simulink model "wheel_leg_backup_621"  (R2025b)
settings: Solver=VariableStepAuto  StartTime=0.0  StopTime=10  FixedStep=0.0001  RelTol=1e-3
undefined symbols (not defined in the file): g, M_L_support, X, Y, Z
libraries: sm_lib x76, nesl_utility x14, slpidlib x1
(part 1 of 3)
settings Model: PauseTimes=10  Creator=Hhop  LastModifiedBy=13422
settings SolverCC: AlgebraicLoopSolver=TrustRegion  MinimalZcImpactIntegration=on
settings DebuggingCC: ReadBeforeWriteMsg=DisableAll  WriteAfterWriteMsg=DisableAll  WriteAfterReadMsg=DisableAll  MultiTaskDSMMsg=none
settings ModelReferenceCC: UpdateModelReferenceTargets=IfOutOfDate
settings SFSimCC: SFSimEcho=off
settings RTWCC: GPUComputeCapability=3.5  DLArmComputeVersion=19.05

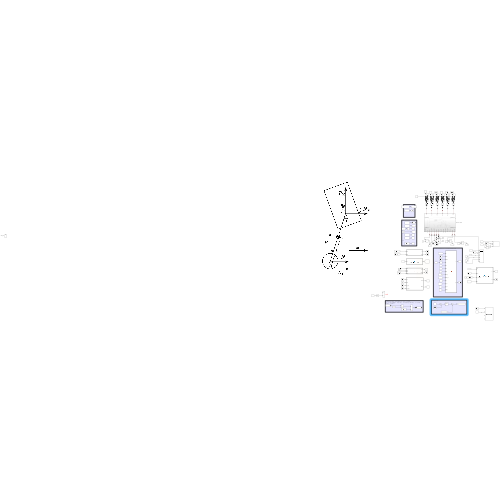
[thumbnail: Simulink's stored preview of the top-level diagram]
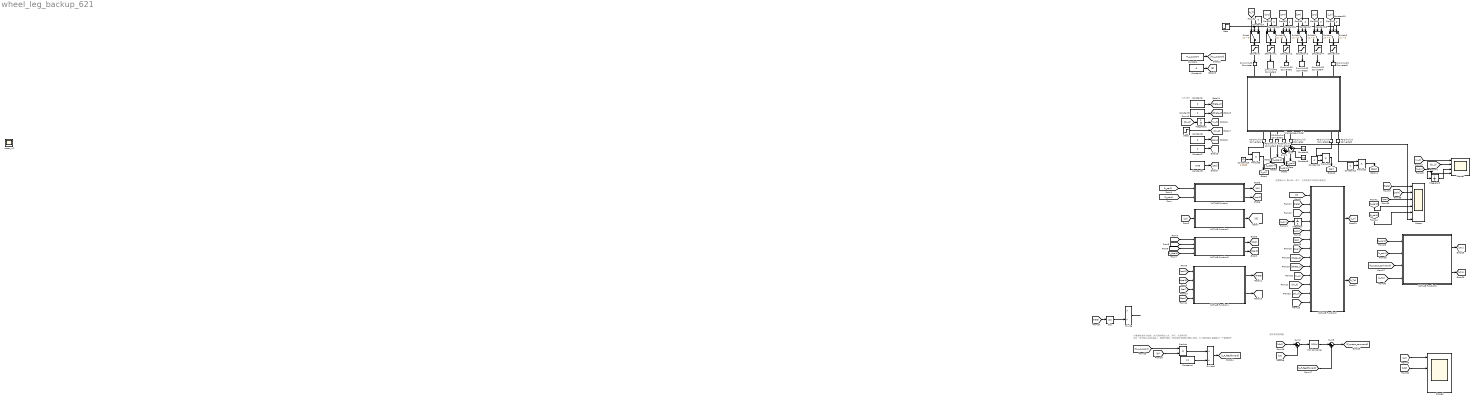
== system wheel_leg_backup_621 ==
  note: 腿长保持控制器
  note: 计算单腿支持力前馈，先只用前馈加上去，开环。之后再闭环.
      | 另外，先不除以costheta了，数值不稳定，而且线性化就是大概在1附近。为了更加稳定
      | 直接除以一个衰减因子
  note: X_d
      |
      |
      |
      |
      |
      |
      |
      |
      |
      |
      |
      |
      |
      |
      |
      |
      |
      |
      | L0d
  note: 这里面dx与x默认RL一样了，之后考虑不对称的时候在改
  Constant : Constant  Value=M_L_support
  Constant1 : Constant  Value=g
  Constant10 : Constant  Value=-1
  Constant11 : Constant  Value=-1
  Constant13 : Constant  Value=0.0603
  Constant{2..3,6..7,14..19} (10 alike) : Constant  Value=0
  Constant4 : Constant  Value=1.2
  Constant5 : Constant  Value=0.08
  Constant8 : Constant  Value=pi/2
  Constant9 : Constant  Value=pi/2
  Cos : Trigonometry  Operator=cos
  Divide : Product  Inputs=*/
  Divide1 : Product  Inputs=*/
  Integrator : Integrator
  Integrator1 : Integrator
  Integrator2 : Integrator
  MATLAB Function : MATLAB Function  TreatAsAtomicUnit=on
  MATLAB Function1 : MATLAB Function  TreatAsAtomicUnit=on
  MATLAB Function2 : MATLAB Function  TreatAsAtomicUnit=on
  MATLAB Function3 : MATLAB Function  TreatAsAtomicUnit=on
  MATLAB Function4 : MATLAB Function  TreatAsAtomicUnit=on
  MATLAB Function5 : MATLAB Function  TreatAsAtomicUnit=on
  PID Controller : slpidlib/PID Controller  Controller=PID  Form=Parallel  TimeDomain=Continuous-time  UseExternalTs=off  SampleTime=-1  IntegratorMethod=Forward Euler  FilterMethod=Forward Euler  ControllerParametersSource=internal  P=220  I=0  UseKiTs=off  D=1000  UseExternalDerivativeSource=off  N=100  UseFilter=on  TunerSelectOption=Transfer Function Based (PID Tuner App)  InitialConditionSource=internal  InitialConditionForIntegrator=0  InitialConditionForFilter=0  DifferentiatorICPrevScaledInput=0  ExternalReset=none  TrackingMode=off  Kt=1  LimitOutput=off  SatLimitsSource=internal  UpperSaturationLimit=inf  LowerSaturationLimit=-inf  LinearizeAsGain=on  AntiWindupMode=none  Kb=1  LimitIntegrator=off  UpperIntegratorSaturationLimit=inf  LowerIntegratorSaturationLimit=-inf  POutMin=[]  POutMax=[]  IOutMin=[]  IOutMax=[]  DOutMin=[]  DOutMax=[]  NOutMin=[]  NOutMax=[]  SumOutMin=[]  SumOutMax=[]  SaturationOutMin=[]  SaturationOutMax=[]  PParamMin=[]  PParamMax=[]  IParamMin=[]  IParamMax=[]  DParamMin=[]  DParamMax=[]  NParamMin=[]  NParamMax=[]  KbParamMin=[]  KbParamMax=[]  KtParamMin=[]  KtParamMax=[]  KbOutMin=[]  KbOutMax=[]  KtOutMin=[]  KtOutMax=[]  IntegratorOutMin=[]  IntegratorOutMax=[]  FilterOutMin=[]  FilterOutMax=[]  SumI1OutMin=[]  SumI1OutMax=[]  SumI2OutMin=[]  SumI2OutMax=[]  SumI3OutMin=[]  SumI3OutMax=[]  SumI4OutMin=[]  SumI4OutMax=[]  SumDOutMin=[]  SumDOutMax=[]  DifferentiatorOutMin=[]  DifferentiatorOutMax=[]  FilterDiffOutCoefMin=[]  FilterDiffOutCoefMax=[]  ReciprocalOutMin=[]  ReciprocalOutMax=[]  SumDenOutMin=[]  SumDenOutMax=[]  SumNumOutMin=[]  SumNumOutMax=[]  DivideOutMin=[]  DivideOutMax=[]  UdiffTsProdOutMin=[]  UdiffTsProdOutMax=[]  NTsProdOutMin=[]  NTsProdOutMax=[]  UintegralTsProdOutMin=[]  UintegralTsProdOutMax=[]  UngainTsProdOutMin=[]  UngainTsProdOutMax=[]  ClampingZeroOutDataTypeStr=Inherit: Inherit via back propagation  ClampingZeroOutMin=[]  ClampingZeroOutMax=[]  FilterDenConstantOutDataTypeStr=Inherit: Inherit via back propagation  FilterDenConstantOutMin=[]  FilterDenConstantOutMax=[]  PCopyOutDataTypeStr=Inherit: Inherit via back propagation  PCopyOutMin=[]  PCopyOutMax=[]  NCopyOutDataTypeStr=Inherit: Inherit via back propagation  NCopyOutMin=[]  NCopyOutMax=[]  IntegratorContinuousStateAttributes=''  IntegratorStateMustResolveToSignalObject=off  IntegratorRTWStateStorageClass=Auto  FilterContinuousStateAttributes=''  FilterStateMustResolveToSignalObject=off  FilterRTWStateStorageClass=Auto  ParallelPVariant=InternalParameters  IdealPVariant=Disabled  IVariant=InternalParameters  DVariant=InternalParameters  IntegratorVariant=Continuous  SatVariant=Disabled  AWVariant=Passthrough  PCopyVariant=Disabled  TRVariant=Disabled  FdbkBlocksVariant=Forward  IdealPFdbkVariant=Disabled  SatFdbkVariant=Disabled  DerivativeFilterVariant=ContFilter  NVariant=InternalParameters  NCopyVariant=Disabled  FilterICVariant=InternalICsFilter  IntegratorICVariant=InternalICs  ExternalResetVariant=Disabled  TRSumVariant=Passthrough  SumFdbkVariant=Disabled  SumVariant=Sum_PID  TsampFilterVariant=InternalTs  TsampNgainVariant=Passthrough  TsampIntegralVariant=Disabled_SignalSpec  ExternalSaturationOutDataTypeStr=Inherit: Same as second input  DerivativeSourceVariant=ErrorSignal  PreIntVariant=InternalPreInt
  PS-Simulink Converter{,1..6} (7 alike) : nesl_utility/PS-Simulink Converter  PhysicalDomain=network_engine_domain  SubClassName=ps_output  LeftPortType=input  RightPortType=output  PseudoPeriodic=off  Frequencies=[]  VectorFormat=inherit  Unit=inherit  AffineConversion=off
  Product{,1..3} (4 alike) : Product
  Saturation : Saturate  UpperLimit=9  LowerLimit=-9
  Saturation{1..4} (4 alike) : Saturate  UpperLimit=100  LowerLimit=-100
  Saturation5 : Saturate  UpperLimit=9  LowerLimit=-9
  Scope : Scope  NumInputPorts=6
      settings: ActiveDisplayYMinimum=-0.39030088912791516  ActiveDisplayYMaximum=1.9087110566025913
  Scope1 : Scope  NumInputPorts=4
      settings: ActiveDisplayYMinimum=-8.4580288493927025  ActiveDisplayYMaximum=9.9670803288475582
  Scope2 : Scope  NumInputPorts=4
      settings: ActiveDisplayYMinimum=-0.42725567392036662  ActiveDisplayYMaximum=0.37749142642233907  DataLoggingVariableName=ScopeData2
  Simulink-PS Converter{,1..5} (6 alike) : nesl_utility/Simulink-PS Converter  PhysicalDomain=network_engine_domain  SubClassName=ps_input  LeftPortType=input  RightPortType=output  PseudoPeriodic=off  Frequencies=[]  NoiseDistribution=none  NoiseParameters=[]  Unit=1  AffineConversion=off  FilteringAndDerivatives=provide  SimscapeFilterOrder=1  InputFilterTimeConstant=0.001  UdotUserProvided=0
  Step : Step  Time=0.2  SampleTime=0
  Step1 : Step  After=0  SampleTime=0
  Sum : Sum  Inputs=|++
  Sum1 : Sum  Inputs=|++
  Sum2 : Sum  Inputs=|+-
  Sum3 : Sum  Inputs=|++
  Switch{,1..5} (6 alike) : Switch  Criteria=u2 > Threshold  SaturateOnIntegerOverflow=off  InputSameDT=off
  blance_leg_model : Subsystem
      settings: PortSchema="{\"entries\":[{\"content\":{\"sides\":[{\"content\":{\"connectorIds\":[\"LConn1\",\"LConn2\",\"LConn3\",\"LConn4\",\"LConn5\",\"LConn6\"]},\"type\":\"ConnectorPlacement.EquallySpacedRectSide\",\"uuid\":\"df2d0b15-ec70-4430-8d90-67c6d88950b4\"},{\"content\":{\"connectorIds\":[\"RConn1\",\"RConn2\",\"RConn3\",\"RConn4\",\"RConn5\",\"RConn6\",\"RConn7\",\"RConn8\",\"RConn9\",\"RConn10\",\"RConn11\",\"RConn12\",\"RConn13\",\"RConn14\"],\"side\":\"RIGHT\"},\"type\":\"ConnectorPlacement.EquallySpacedRectSide\",\"uuid\":\"ec9b4787-d265-4ad9-b676-e253d2304993\"},{\"content\":{\"connectorIds\":[\"LConn7\",\"LConn8\"],\"side\":\"TOP\"},\"type\":\"ConnectorPlacement.EquallySpacedRectSide\",\"uuid\":\"40dd08fe-dc32-4cee-bbb8-c1ec6d04ee32\"},{\"content\":{\"connectorIds\":[\"RConn15\",\"RConn16\"],\"side\":\"BOTTOM\"},\"type\":\"ConnectorPlacement.EquallySpacedRectSide\",\"uuid\":\"0f9c1faf-3e52-4dca-bbb1-0993be9fa88c\"}]},\"type\":\"ConnectorPlacement.EquallySpacedConnector\",\"uuid\":\"d540d646-85aa-4f97-ae4d-1bccec971368\"}],\"packageUris\":[\"http://schema.mathworks.com/mf0/Connector/R2020b\"],\"version\":\"1.0\"}"
  mean_x2 : Scope
      settings: ActiveDisplayYMinimum=-0.05008  ActiveDisplayYMaximum=0.21605  DataLoggingVariableName=ScopeData16
  wires:
  Sum/1 -> [L_pai4]
  PS-Simulink Converter2/1 -> [L_dpai1]
  PS-Simulink Converter4/1 -> Product3/1
  PS-Simulink Converter1/1 -> [L_dpai4]
  [L_pai4] -> MATLAB Function/2(pai4)
  [L_pai1] -> MATLAB Function/1(pai1)
  MATLAB Function/1(L0) -> [L0]
  MATLAB Function/2(pai0) -> [pai0]
  [L0] -> MATLAB Function1/1(L0)
  MATLAB Function1/1(K) -> [K]
  [K] -> MATLAB Function2/1(K)
  [L_pai1] -> MATLAB Function3/1(phi1)
  [L_pai4] -> MATLAB Function3/2(phi4)
  [L_dpai1] -> MATLAB Function3/3(dphi1)
  [L_dpai4] -> MATLAB Function3/4(dphi4)
  MATLAB Function3/1(dL0) -> [dL0]
  MATLAB Function3/2(dphi0) -> [dpai0]
  [pai0] -> MATLAB Function4/1(phi0)
  [dpai0] -> MATLAB Function4/2(dphi0)
  PS-Simulink Converter6/1 -> Product1/1
  PS-Simulink Converter5/1 -> Product2/1
  [pai] -> MATLAB Function4/3(body_phi)
  [dpai] -> MATLAB Function4/4(body_dphi)
  MATLAB Function4/2(dtheta) -> [dtheta]
  MATLAB Function4/1(theta) -> [theta]
  [dtheta] -> MATLAB Function2/3(dtheta)
  [L_dx] -> MATLAB Function2/5(dx)
  Integrator/1 -> MATLAB Function2/4(x)
  [L_dx] -> Integrator/1
  [pai] -> MATLAB Function2/6(phi)
  [dpai] -> MATLAB Function2/7(dphi)
  [theta] -> MATLAB Function2/2(theta)
  Constant2/1 -> [theta_d]
  Constant3/1 -> [dtheta_d]
  Integrator1/1 -> [x_d]
  Step1/1 -> [dx_d]
  Constant6/1 -> [pai_d]
  Constant7/1 -> [dpai_d]
  [theta_d] -> MATLAB Function2/8(theta_d)
  [dtheta_d] -> MATLAB Function2/9(dtheta_d)
  [x_d] -> MATLAB Function2/10(x_d)
  [dx_d] -> MATLAB Function2/11(dx_d)
  [pai_d] -> MATLAB Function2/12(phi_d)
  [dpai_d] -> MATLAB Function2/13(dphi_d)
  MATLAB Function2/1(T) -> [L_T]
  MATLAB Function2/2(Tp) -> [L_Tp]
  [theta] -> Cos/1
  Cos/1 -> Divide/2
  Constant/1 -> [M_L_support]
  Constant1/1 -> [g]
  [M_L_support] -> Product/1
  [g] -> Product/2
  Divide/1 -> ?
  [L_pai1] -> MATLAB Function5/1(phi1)
  [L_pai4] -> MATLAB Function5/2(phi4)
  [L_Tp] -> MATLAB Function5/4(Tp)
  MATLAB Function5/1(T1) -> [LT1]
  MATLAB Function5/2(T4) -> [LT4]
  [theta] -> Scope/1  "theta"
  [pai0] -> Scope/2  "pai0"
  [pai] -> Scope/3  "pai"
  PS-Simulink Converter3/1 -> Sum1/1
  Sum1/1 -> [L_pai1]
  [L_pai1] -> Scope/4  "pai1"
  [L_pai4] -> Scope/5  "pai4"
  PS-Simulink Converter/1 -> Scope/6, Sum/1
  Constant8/1 -> Sum1/2
  Constant9/1 -> Sum/2
  Constant10/1 -> Product1/2
  Product1/1 -> [pai]
  Constant11/1 -> Product2/2
  Product2/1 -> [dpai]
  Saturation2/1 -> Simulink-PS Converter2/1
  Saturation5/1 -> Simulink-PS Converter5/1
  Saturation3/1 -> Simulink-PS Converter3/1
  [L_T] -> Switch/1
  Saturation1/1 -> Simulink-PS Converter1/1
  Saturation4/1 -> Simulink-PS Converter4/1
  Saturation/1 -> Simulink-PS Converter/1
  Constant13/1 -> Product3/2
  Product3/1 -> [L_dx]
  Constant14/1 -> Switch/3
  Switch/1 -> Saturation/1
  Constant15/1 -> Switch1/3
  [LT1] -> Switch1/1
  Constant16/1 -> Switch2/3
  [LT4] -> Switch2/1
  Constant17/1 -> Switch3/3
  [LT4] -> Switch3/1
  Constant18/1 -> Switch4/3
  [LT1] -> Switch4/1
  Constant19/1 -> Switch5/3
  [L_T] -> Switch5/1
  Switch1/1 -> Saturation1/1
  Switch2/1 -> Saturation2/1
  Switch3/1 -> Saturation3/1
  Switch4/1 -> Saturation4/1
  Switch5/1 -> Saturation5/1
  Step/1 -> Switch/2, Switch5/2, Switch4/2, Switch3/2, Switch2/2, Switch1/2
  [F_output_command] -> MATLAB Function5/3(F_command)
  [dx_d] -> Integrator1/1
  [x_d] -> Scope1/1  "xd"
  [dx_d] -> Scope1/2  "dxd"
  [L_dx] -> Scope1/4, Integrator2/1  "dx"
  Integrator2/1 -> Scope1/3  "x"
  Product/1 -> Divide1/1
  Constant4/1 -> Divide1/2
  Constant5/1 -> [L0d]
  Sum2/1 -> PID Controller/1
  [L0d] -> Sum2/1
  PID Controller/1 -> Sum3/1
  [L_F_feedforward] -> Sum3/2
  [L0] -> Sum2/2
  Sum3/1 -> [F_output_command]
  [L0] -> Scope2/1  "L0"
  [L0d] -> Scope2/2  "L0d"
  Divide1/1 -> [L_F_feedforward]
  connections:
  blance_leg_model/RConn7 -- PS-Simulink Converter/LConn1
  PS-Simulink Converter1/LConn1 -- blance_leg_model/RConn4
  PS-Simulink Converter2/LConn1 -- blance_leg_model/RConn5
  PS-Simulink Converter4/LConn1 -- blance_leg_model/RConn3
  blance_leg_model/RConn6 -- PS-Simulink Converter3/LConn1
  PS-Simulink Converter5/LConn1 -- blance_leg_model/RConn14
  PS-Simulink Converter6/LConn1 -- blance_leg_model/RConn13
  blance_leg_model/LConn2 -- Simulink-PS Converter1/RConn1
  blance_leg_model/LConn4 -- Simulink-PS Converter3/RConn1
  blance_leg_model/LConn1 -- Simulink-PS Converter/RConn1
  blance_leg_model/LConn3 -- Simulink-PS Converter2/RConn1
  blance_leg_model/LConn5 -- Simulink-PS Converter4/RConn1
  blance_leg_model/LConn6 -- Simulink-PS Converter5/RConn1
